simulink model "feedback_yd"  (R2022b)
settings: Solver=VariableStepAuto  StartTime=0.0  StopTime=10.0  RelTol=1e-3
model workspace (MAT data in the model file):
  k1 = Simulink.Parameter
  k1.Value = 30
  k1.DataType = 'auto'
  k1.Complexity = 'real'
  k1.Dimensions = [1 1]
  k2 = Simulink.Parameter
  k2.Value = 1.5
  k2.DataType = 'auto'
  k2.Complexity = 'real'
  k2.Dimensions = [1 1]
libraries: robotmobilelib x1
settings Model: Creator=thoma  LastModifiedBy=thoma

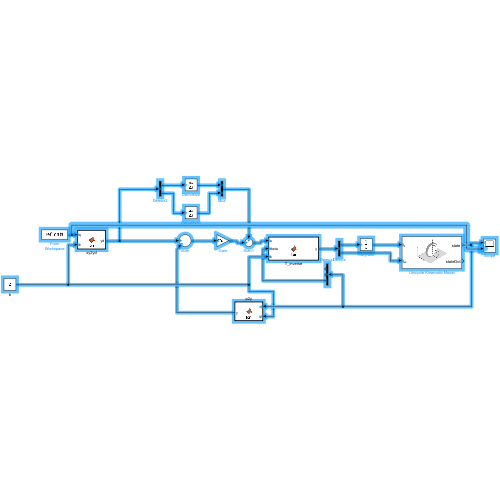
[thumbnail: Simulink's stored preview of the top-level diagram]
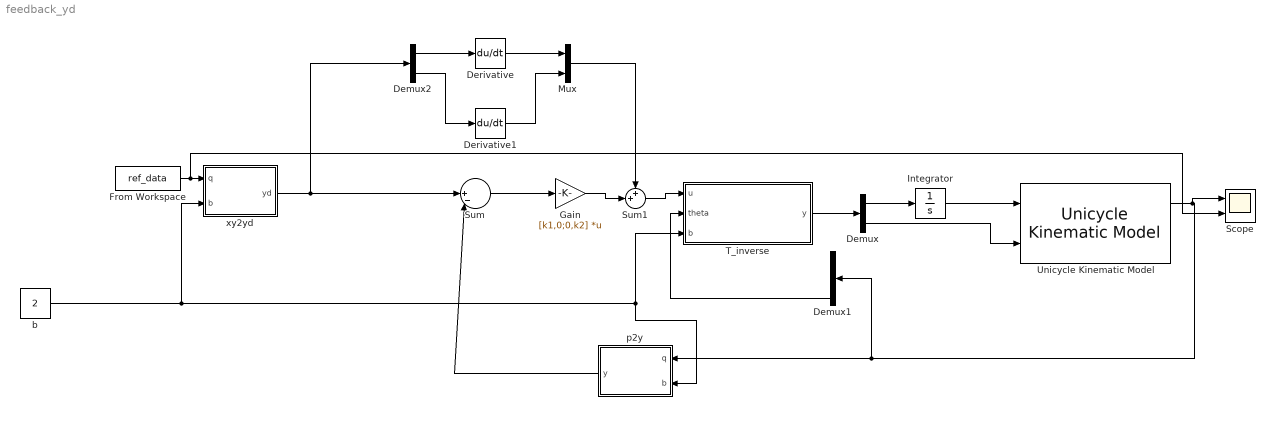
== system feedback_yd ==
  Demux : Demux  Outputs=2
  Demux1 : Demux  Outputs=3
  Demux2 : Demux  Outputs=2
  Derivative : Derivative
  Derivative1 : Derivative
  From Workspace : FromWorkspace  VariableName=ref_data
  Gain : Gain  Gain=[k1,0;0,k2]  Multiplication=Matrix(K*u)
  Integrator : Integrator
  Mux : Mux  Inputs=2
  Scope : Scope  NumInputPorts=2
  Sum : Sum  Inputs=||+-|
  Sum1 : Sum  Inputs=++|
  T_inverse : MATLAB Function  TreatAsAtomicUnit=on
  Unicycle Kinematic Model : robotmobilelib/Unicycle Kinematic Model  VehicleInputs=Vehicle Speed & Heading Angular Velocity  WheelRadius=2  WheelSpeedRange=[-Inf Inf]  InitialState=[0; 0; 0]  SimulateUsing=Interpreted execution
  b : Constant  Value=2
  p2y : MATLAB Function  TreatAsAtomicUnit=on
  xy2yd : MATLAB Function  TreatAsAtomicUnit=on
  wires:
  T_inverse/1(y) -> Demux/1
  Demux/2 -> Unicycle Kinematic Model/2
  Demux1/3 -> T_inverse/2(theta)
  p2y/1(y) -> Sum/2
  Sum1/1 -> T_inverse/1(u)
  Unicycle Kinematic Model/1 -> Scope/1, Demux1/1, p2y/1(q)
  Demux/1 -> Integrator/1
  Integrator/1 -> Unicycle Kinematic Model/1
  b/1 -> xy2yd/2(b), T_inverse/3(b), p2y/2(b)
  Sum/1 -> Gain/1
  Gain/1 -> Sum1/2
  From Workspace/1 -> Scope/2, xy2yd/1(q)
  xy2yd/1(yd) -> Demux2/1, Sum/1
  Demux2/1 -> Derivative/1
  Derivative/1 -> Mux/1
  Demux2/2 -> Derivative1/1
  Derivative1/1 -> Mux/2
  Mux/1 -> Sum1/1

== matlab function feedback_yd/T_inverse ==
  data: u input; y output; theta input; b input
function y = fcn(u,theta,b)
T_inverse=[cos(theta),sin(theta);-sin(theta)/b,cos(theta)/b];
vet=T_inverse*u;
a=vet(1);
w=vet(2);
y = vet;

== matlab function feedback_yd/xy2yd ==
  data: q input; yd output; b input
function yd = fcn(q,b)
x=q(1);
y=q(2);
theta=q(3);
y1=x+b*cos(theta);
y2=y+b*sin(theta);
yd=[y1;y2];

== matlab function feedback_yd/p2y ==
  data: q input; y output; b input
function y = fcn(q,b)
x=q(1);
yi=q(2);
theta=q(3);
y1=x+b*cos(theta);
y2=yi+b*sin(theta);
y=[y1;y2];
